simulink model "momentumBasedFlying"  (R2021b)
settings: Solver=FixedStepAuto  StartTime=0.0  StopTime=Config.simulationTime  FixedStep=Config.tStep  RelTol=1e-3
InitFcn:
  | cd(fileparts(which(bdroot)));
  | initMomentumBasedFlying;
StopFcn:
  | cd(fileparts(which(bdroot)));
  | stopMomentumBasedFlying;
undefined symbols (not defined in the file or in its folder): biasVectorConstraint_feet, Config, confVisualizer, ConstraintMatrix_feet, DiscIntNeverNeededParam, jets_config
libraries: WBToolboxLibrary x75
(part 4 of 4)

== matlab function momentumBasedFlying/FLYING CONTROLLER (CORE) V2.5/Flight Controller RAL-HUMANOIDS V3.1- Aerodynamic Effects Compensation/Momentum Control for Flying/QP Solver and Integrate Contact Forces Derivative/Integrate the Contact Forces Derivative/deadZone/Deadzone Function ==
  data: u input; y output; thr input
function y = deadZoneFCN(u, thr)

    y = wbc.deadZone(u, thr);
end

== matlab function momentumBasedFlying/FLYING CONTROLLER (CORE) V2.5/Flight Controller RAL-HUMANOIDS V3.1- Aerodynamic Effects Compensation/Momentum Control for Flying/QP Solver and Integrate Contact Forces Derivative/QP momentumControl/Process QP Inputs Momentum Control ==
  data: HessianMatrixQP input; H_balancing output; gVectorQP input; lowerBoundQP input; upperBoundQP input; g_balancing output; ub_balancing output; lb_balancing output; H_flight output; g_flight output; ub_flight output; lb_flight output
function [H_balancing,g_balancing,ub_balancing,lb_balancing, ...
          H_flight,g_flight,ub_flight,lb_flight] = processQPinputMomentumControlFCN(HessianMatrixQP,gVectorQP,lowerBoundQP,upperBoundQP) 
      
    [H_balancing,g_balancing,ub_balancing,lb_balancing, ...
        H_flight,g_flight,ub_flight,lb_flight] = iRonCubLib.processQPinputMomentumControl(HessianMatrixQP,gVectorQP,lowerBoundQP,upperBoundQP);
end

== matlab function momentumBasedFlying/FLYING CONTROLLER (CORE) V2.5/Flight Controller RAL-HUMANOIDS V3.1- Aerodynamic Effects Compensation/Momentum Control for Flying/Feedback linearization/MATLAB Function ==
  data: jets input; jets_dot input; jets_dot_des input; throttle output size=[4,1]; Config parameter; error output; integral_err input
function [throttle, error]  = fl_jet_control(jets, jets_dot, jets_dot_des, Config, integral_err)

[throttle, error]  = fl_jet_control(jets, jets_dot, jets_dot_des, Config, integral_err);
end

== matlab function momentumBasedFlying/FLYING CONTROLLER (CORE) V2.5/Flight Controller RAL-HUMANOIDS V3.1- Aerodynamic Effects Compensation/Momentum Control for Flying/extendedKalmanFilter4jets/EKF_jet1/EKF  ==
  data: x input; input input; measurement input; xDot output; P input; Config parameter; Pdot output
function [xDot, Pdot] = extendedKalmanFilterFNC(x, input, measurement, P, Config)

[xDot, Pdot] = extKalmanFilter(x, input, Config.jetC_P100, P, measurement, Config);

== matlab function momentumBasedFlying/FLYING CONTROLLER (CORE) V2.5/Flight Controller RAL-HUMANOIDS V3.1- Aerodynamic Effects Compensation/Momentum Control for Flying/extendedKalmanFilter4jets/EKF_jet1/splitVector ==
  data: x input; x1 output; x2 output
function [x1, x2] = fcn(x)
x1 = x(1);
x2 = x(2);

== matlab function momentumBasedFlying/FLYING CONTROLLER (CORE) V2.5/Flight Controller RAL-HUMANOIDS V3.1- Aerodynamic Effects Compensation/Momentum Control for Flying/extendedKalmanFilter4jets/EKF_jet2/EKF  ==
  data: x input; input input; measurement input; xDot output; P input; Config parameter; Pdot output
function [xDot, Pdot] = extendedKalmanFilterFNC(x, input, measurement, P, Config)

[xDot, Pdot] = extKalmanFilter(x, input, Config.jetC_P100, P, measurement, Config);

== matlab function momentumBasedFlying/FLYING CONTROLLER (CORE) V2.5/Flight Controller RAL-HUMANOIDS V3.1- Aerodynamic Effects Compensation/Momentum Control for Flying/extendedKalmanFilter4jets/EKF_jet2/splitVector ==
  data: x input; x1 output; x2 output
function [x1, x2] = fcn(x)
x1 = x(1);
x2 = x(2);

== matlab function momentumBasedFlying/FLYING CONTROLLER (CORE) V2.5/Flight Controller RAL-HUMANOIDS V3.1- Aerodynamic Effects Compensation/Momentum Control for Flying/extendedKalmanFilter4jets/EKF_jet3/EKF  ==
  data: x input; input input; measurement input; xDot output; P input; Config parameter; Pdot output
function [xDot, Pdot] = extendedKalmanFilterFNC(x, input, measurement, P, Config)

[xDot, Pdot] = extKalmanFilter(x, input, Config.jetC_P220, P, measurement, Config);

== matlab function momentumBasedFlying/FLYING CONTROLLER (CORE) V2.5/Flight Controller RAL-HUMANOIDS V3.1- Aerodynamic Effects Compensation/Momentum Control for Flying/extendedKalmanFilter4jets/EKF_jet3/splitVector ==
  data: x input; x1 output; x2 output
function [x1, x2] = fcn(x)
x1 = x(1);
x2 = x(2);

== matlab function momentumBasedFlying/FLYING CONTROLLER (CORE) V2.5/Flight Controller RAL-HUMANOIDS V3.1- Aerodynamic Effects Compensation/Momentum Control for Flying/extendedKalmanFilter4jets/EKF_jet4/EKF  ==
  data: x input; input input; measurement input; xDot output; P input; Config parameter; Pdot output
function [xDot, Pdot] = extendedKalmanFilterFNC(x, input, measurement, P, Config)

[xDot, Pdot] = extKalmanFilter(x, input, Config.jetC_P220, P, measurement, Config);

== matlab function momentumBasedFlying/FLYING CONTROLLER (CORE) V2.5/Flight Controller RAL-HUMANOIDS V3.1- Aerodynamic Effects Compensation/Momentum Control for Flying/extendedKalmanFilter4jets/EKF_jet4/splitVector ==
  data: x input; x1 output; x2 output
function [x1, x2] = fcn(x)
x1 = x(1);
x2 = x(2);

== matlab function momentumBasedFlying/Visualizer/Task and Base Frame Kinematics/MATLAB Function1 ==
  data: RPY_Corr output; rollPitchYaw input
function RPY_Corr = correctYawAngleFCN(rollPitchYaw)

    RPY_Corr = correctYawAngle(rollPitchYaw);

end

== matlab function momentumBasedFlying/Visualizer/Task and Base Frame Kinematics/MATLAB Function3 ==
  data: RPY_Corr output; rollPitchYaw input
function RPY_Corr = correctYawAngleFCN(rollPitchYaw)

    RPY_Corr = correctYawAngle(rollPitchYaw);

end
